simulink model "non_linear_Position_System_control101"  (R2023b)
settings: Solver=ode45  StartTime=0.0  StopTime=endtime  RelTol=1e-3  EnableMultiTasking=on
undefined symbols (not defined in the file): backlashonoff, C, d, Dumax, Dumin, km, ks, measurementdelay, P, R, saturationonoff, umax, umin
settings Model: Creator=stelios  LastModifiedBy=Anthony Rossiter
settings DataIOCC: LimitDataPoints=on  SaveFormat=Array  SignalLoggingSaveFormat=ModelDataLogs  ReturnWorkspaceOutputs=off
settings OptimizationCC: BooleanDataType=off
settings DebuggingCC: SaveWithParameterizedLinksMsg=none  UnderspecifiedInitializationDetection=Classic  MergeDetectMultiDrivingBlocksExec=none  SignalResolutionControl=TryResolveAllWithWarning  InheritedTsInSrcMsg=none  MultiTaskDSMMsg=warning  MultiTaskCondExecSysMsg=none  UnconnectedInputMsg=warning  UnconnectedOutputMsg=warning  UnconnectedLineMsg=warning
settings HardwareCC: TargetUnknown=on
settings ModelReferenceCC: EnableRefExpFcnMdlSchedulingChecks=on  PropagateSignalLabelsOutOfModel=off
settings RTWCC: DLArmComputeVersion=19.05
settings GRTTargetCC: CombineOutputUpdateFcns=off  GRTInterface=on
settings ConfigComp: CovMetricSettings=dw

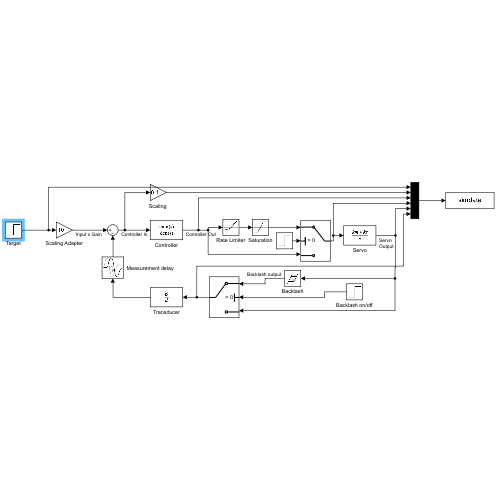
[thumbnail: Simulink's stored preview of the top-level diagram]
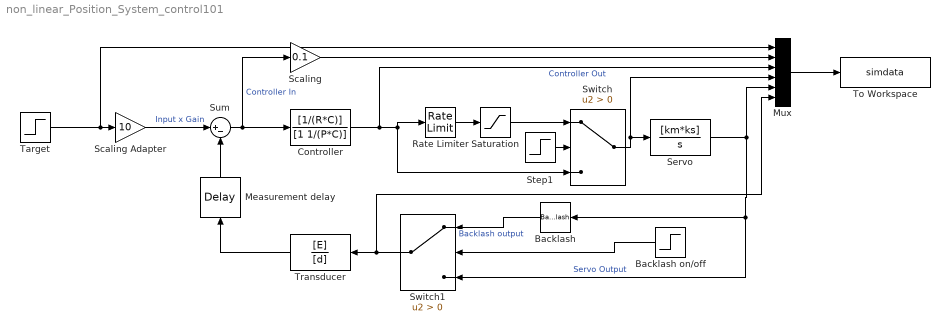
== system non_linear_Position_System_control101 ==
  Backlash : Backlash  BacklashWidth=deadband
  Backlash on/off : Step  Time=0  After=backlashonoff
  Controller : TransferFcn  Numerator=[1/(R*C)]  Denominator=[1 1/(P*C)]
  Measurement delay : TransportDelay  DelayTime=measurementdelay  TransDelayFeedthrough=on
  Mux : Mux  Inputs=6
  Rate Limiter : RateLimiter  RisingSlewLimit=Dumax  FallingSlewLimit=Dumin  SampleTimeMode=inherited
  Saturation : Saturate  UpperLimit=umax  LowerLimit=umin
  "Scaling " : Gain  Gain=0.1  SaturateOnIntegerOverflow=on
  Scaling Adapter : Gain  Gain=10  SaturateOnIntegerOverflow=on
  Servo : TransferFcn  Numerator=[km*ks]  Denominator=[1 0]
  Step1 : Step  Time=0  After=saturationonoff
  Sum : Sum  Inputs=|+-  SaturateOnIntegerOverflow=on
  Switch : Switch  Criteria=u2 > Threshold  SaturateOnIntegerOverflow=off  InputSameDT=off
  Switch1 : Switch  Criteria=u2 > Threshold  SaturateOnIntegerOverflow=off  InputSameDT=off
  Target : Step  Time=0.2  After=1.3
  To Workspace : ToWorkspace  VariableName=simdata  SaveFormat=Structure With Time  SampleTime=-1
  Transducer : TransferFcn  Numerator=[E]  Denominator=[d]
  wires:
  Sum/1 -> "Scaling "/1, Controller/1  "Controller In"
  Servo/1 -> Mux/5, Switch1/3, Backlash/1  "Servo Output"
  Transducer/1 -> Measurement delay/1
  Target/1 -> Mux/1, Scaling Adapter/1
  Scaling Adapter/1 -> Sum/1  "Input x Gain"
  Controller/1 -> Switch/3, Rate Limiter/1, Mux/3  "Controller Out"
  Mux/1 -> To Workspace/1
  Switch/1 -> Mux/4, Servo/1
  Saturation/1 -> Switch/1
  Rate Limiter/1 -> Saturation/1
  Step1/1 -> Switch/2
  Backlash/1 -> Switch1/1  "Backlash output"
  Backlash on/off/1 -> Switch1/2
  Switch1/1 -> Mux/6, Transducer/1
  "Scaling "/1 -> Mux/2
  Measurement delay/1 -> Sum/2
